simulink model "Task1"  (R2025a)
settings: Solver=VariableStepAuto  StartTime=0.0  StopTime=10.0  RelTol=1e-3
values from neighbouring files (symbols this model uses):
  EbNo_val = 10    [init_params.m]    (also in run_simulation.m = EbNo_Range(i))
  k = 4    [Script.m]    (also in Script_task1.m; Script_task12_mix.m; Script_task1_HyperModulation.m; Script_task3.m)
  SymbolRate = Fs/Sps    (= 25000)    [init_params.m]    (also in run_simulation.m = 1000)
libraries: commdigbbndpm3 x2, commchan3 x1, commrandsrc3 x1, commsink2 x1
settings Model: Creator=danie  LastModifiedBy=danie

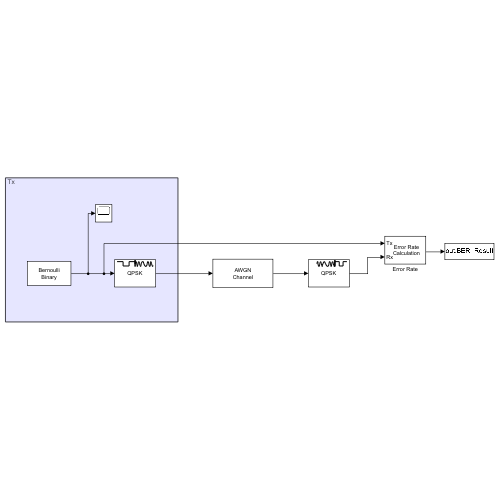
[thumbnail: Simulink's stored preview of the top-level diagram]
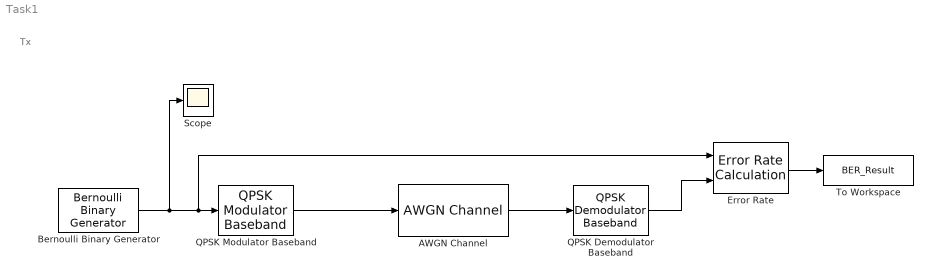
== system Task1 ==
  note: Tx
  AWGN Channel : commchan3/AWGN Channel  LegacyMode=off  NoiseMethod="Signal to noise ratio  (SNR)"  noiseMode="Signal to noise ratio  (SNR)"  EbNo=100  EsNo=10  SNR=EbNo_val + 10*log10(k)  BitsPerSymbol=1  SignalPower=1  SpecifySymbolPeriod=on  SamplesPerSymbol=1  SymbolPeriod=1/SymbolRate  VarianceSource=Parameter  Variance=1  RandomStream=Global stream  Seed=67  SimulateUsing=Code generation
  Bernoulli Binary Generator : commrandsrc3/Bernoulli Binary Generator  ProbabilityOfZero=0.5  SeedSource=Auto  Seed=0  SampleTime=k/SymbolRate  SamplesPerFrame=k  OutputDataType=double  SimulateUsing=Interpreted execution
  Error Rate : commsink2/Error Rate Calculation  N=0  st_delay=0  cp_mode=Entire frame  subframe=[]  PMode=Port  WsName=ErrorVec  RsMode2=off  stop=off  numErr=100  maxBits=1e6
  QPSK Demodulator Baseband : commdigbbndpm3/QPSK Demodulator Baseband  OutType=Bit  DecType=Hard decision  VarSource=Dialog  Variance=1  Dec=Gray  Ph=pi/4  outDtype1=Inherit via internal rule  outDtype2=Inherit via internal rule  derotateFactorWordLen=16  derotateFactorDataTypeStr=Inherit: Same word length as input  derotateFactorLastDataTypeStr=Inherit: Same word length as input
  QPSK Modulator Baseband : commdigbbndpm3/QPSK Modulator Baseband  InType=Bit  Enc=Gray  Ph=pi/4  outDtype=double  outWordLen=16  outUDDataType=sfix(16)  outFracLenMode=Best precision  outFracLen=15  outDataTypeStr=double  outLastDataTypeStr=double
  Scope : Scope
      settings: ActiveDisplayYMinimum=-0.037147900380229415  ActiveDisplayYMaximum=0.94225980770534457
  To Workspace : ToWorkspace  VariableName=BER_Result  SampleTime=-1
  wires:
  Bernoulli Binary Generator/1 -> Scope/1, Error Rate/1, QPSK Modulator Baseband/1
  QPSK Modulator Baseband/1 -> AWGN Channel/1
  AWGN Channel/1 -> QPSK Demodulator Baseband/1
  Error Rate/1 -> To Workspace/1
  QPSK Demodulator Baseband/1 -> Error Rate/2
